simulink model "main_vehicle_v2"  (R2024b)
settings: Solver=FixedStepAuto  StartTime=0.0  StopTime=20  FixedStep=Ts  RelTol=1e-3
values from neighbouring files (symbols this model uses):
  Frr = Crr*m*g    (= 53.955)    [main_data_vehicle.m]
  v0 = 0.1    [main_data_vehicle.m]
undefined symbols (not defined in the file or in its folder): Sim3dSensor
libraries: sim3dlib x3, simulink x2, sim3dautolib x1, dspvision x1
settings Model: Creator=marti  LastModifiedBy=marti

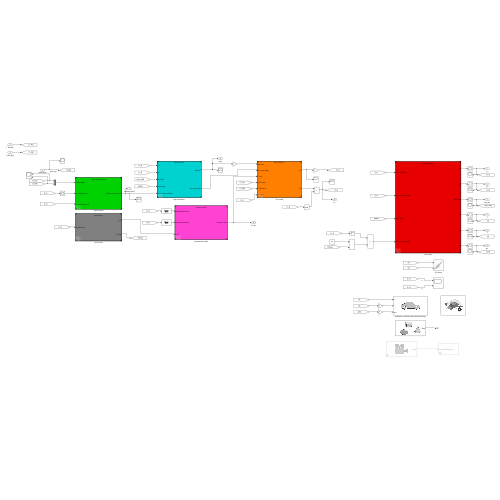
[thumbnail: Simulink's stored preview of the top-level diagram]
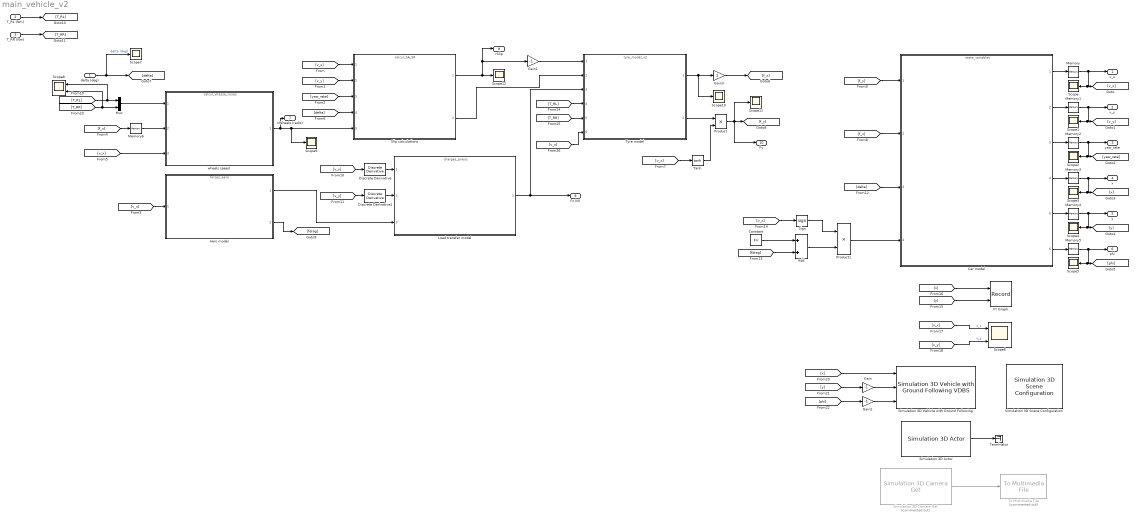
== system main_vehicle_v2 ==
  delta (deg) : Inport
  T_RL (Nm) : Inport  Port=2
  T_RR (Nm) : Inport  Port=3
  Add : Sum
  Aero model : ModelReference  ModelNameDialog=forces_aero.slx  SimulationMode=Normal  ModelReferenceVersion=1.5
  Car model : ModelReference  ModelNameDialog=state_variables.slx  SimulationMode=Normal  ModelReferenceVersion=1.11
  Constant : Constant  Value=Frr
  Discrete Derivative : simulink/Discrete/Discrete Derivative  gainval=1.0  ICPrevScaledInput=0.0  OutMin=[]  OutMax=[]  OutDataType=fixdt(1, 16)  OutScaling=2^-10  DoSatur=off
  Discrete Derivative1 : simulink/Discrete/Discrete Derivative  gainval=1.0  ICPrevScaledInput=0.0  OutMin=[]  OutMax=[]  OutDataType=fixdt(1, 16)  OutScaling=2^-10  DoSatur=off
  Gain : Gain  Gain=-1
  Gain1 : Gain  Gain=-1
  Gain2 : Gain  Gain=-1
  Gain3 : Gain
  Load transfer model : ModelReference  ModelNameDialog=charges_pneus.slx  SimulationMode=Normal  ModelReferenceVersion=1.22
  Memory : Memory  InitialCondition=v0
  Memory{1..5} (5 alike) : Memory
  Memory6 : Memory  InitialCondition=[0 0 0 0]
  Mux : Mux  Inputs=2
  Product : Product
  Product1 : Product
  Scope{,1..5,7,9..12} (11 alike) : Scope
  Scope6 : Scope  NumInputPorts=2
  Scope8 : Scope  NumInputPorts=2
  Sign : Signum
  Simulation 3D Actor : sim3dlib/Simulation 3D Actor  ActorName=Sim3dActor5  ParentName=Scene Origin  Operation=Create at setup  InitScriptText=skidpadConePlacement  SampleTime=.03  Translation=single([0 0 0])  Rotation=single([0 0 0])  Scale=single([1 1 1])  aMode=5  ActorTag=Sim3dActor5  ActorType=Sim3dActor  ID=5
      settings: LibrarySourceBlock=sl3dlib/Simulation 3D/Simulation 3D Actor
  Simulation 3D Camera Get : sim3dlib/Simulation 3D Camera Get  Priority=1  Commented=on  sensorTag=Sim3dSensor�  sensorId=2  sensorName=Sim3dSensor�  vehTagList={'Scene Origin';'Sim3dActor1';'Sim3dActor2';'Sim3dActor3';'Sim3dActor4';'Sim3dActor5';'SimulinkVehicle1'}  vehTag=SimulinkVehicle1  mountLoc=Origin  offsetFlag=on  tmountOffset=[-8, 0, 1]  rmountOffset=[0, 0, 0]  HorizontalResolution=1280  VerticalResolution=720  HorizontalFOV=60  SampleTime=0.03  mountPoint=[-8 0 1]  mountOrientation=[0 0 0]  aMode=5  ID=2
      settings: LibrarySourceBlock=sl3dlib/Simulation 3D/Utilities/Simulation 3D Camera Get
  Simulation 3D Scene Configuration : sim3dlib/Simulation 3D Scene Configuration  Priority=0  ProjectFormat=Default Scenes  SceneDesc=Straight road  ProjectName=C:\Program Files\MATLAB\R2024b\toolbox\shared\sim3d_projects\automotive_project_windows\UE\WindowsNoEditor\VehicleSimulation.exe  ScenePath=/Game/Maps/HwStrght  EnableOpenDRIVE=off  vehTagList={'Custom';'Scene Origin';'Sim3dActor1';'Sim3dActor2';'Sim3dActor3';'Sim3dActor4';'Sim3dActor5';'SimulinkVehicle1'}  vehTag=SimulinkVehicle1  FreeCameraInitialTranslation=[0, 0, 0]  FreeCameraDefaultInitialTranslation=[-6, 0, 2]  FreeCameraInitialRotation=[0, 0, 0]  FreeCameraDefaultInitialRotation=[0, -15, 0]  OpVisEn=off  Ts=.03  EnableWindow=on  EnableRemoteAccess=off  EnableWeather=off  SunAzimuth=90  SunAltitude=40.0  EnableGeospatialSun=off  Latitude=0  Longitude=0  Date=2023-01-01  Time=10:30:00  GeoTimeZone=-5.0  SunDaylightSaving=off  wind=1  clouds=10  EnableVolumetricClouds=off  CloudCoverage=0  CloudAltitude=6  fog=0  rain=0  RaindropsEffect=off  SnowDensity=0  EnableGeospatial=off  UseTrueOrigin=off  OriginHeight=200  OriginLatitude=40.744652  OriginLongitude=-73.988864  MapStyle=Aerial  AdditionalAssetIDs=[]  UseAdvancedSunSky=off  SolarTime=11  TimeZone=-5  Day=21  Month=9  Year=2022  UseDaylightSavingTime=on  DSTStartDay=10  DSTStartMonth=3  DSTEndDay=3  DSTEndMonth=11  DSTSwitchHour=2  sensorTag=MainCamera1  sensorId=1  sensorName=MainCamera1  mountLoc=Origin  offsetFlag=off  tmountOffset=[0, 0, 0]  rmountOffset=[0, 0, 0]  HorizontalResolution=1280  VerticalResolution=720  HorizontalFOV=60  mountPoint=[0 0 0]  mountOrientation=[0 0 0]  aMode=2  ID=1  GeoTrigger=Inactive
      settings: LibrarySourceBlock=vehdynlibsim3dcore/Simulation 3D Scene Configuration
  Simulation 3D Vehicle with Ground Following : sim3dautolib/Simulation 3D Vehicle with Ground Following VDBS  Priority=-1  PassVehMesh=Formula student vehicle  MeshPath=/MathWorksAutomotiveContent/Vehicles/Muscle/Meshes/SK_MuscleCar.SK_MuscleCar  TrackWidth=1.9  WheelBase=3  WheelRadius=0.35  VehColor=Silver  InitialPos=[0, 0, 0]  InitialRot=[0, 0, 0]  ActorName=SimulinkVehicle1  VehLightsControl=off  HeadlightColor=[ 1, 1, 1 ]  HighBeamIntensity=100000  LowBeamIntensity=60000  HighBeamConeAngle=1.22  LowBeamConeAngle=1.22  LeftHeadlightOrientation=[ 0, 0 ]  RightHeadlightOrientation=[ 0, 0 ]  BrakelightIntensity=200  ReverselightIntensity=500  SignallightIntensity=500  SignallightPeriod=1  SignalPulseWidth=50  SampleTime=-1  ActorType=SimulinkVehicle  ID=1  aMode=2  ActorTag=SimulinkVehicle1  CoordinateScheme=SAE
      settings: LibrarySourceBlock=vehdynlibsim3d/Simulation 3D Vehicle with Ground Following
  Slip calculations : ModelReference  ModelNameDialog=calcul_SA_SR.slx  SimulationMode=Normal  ModelReferenceVersion=1.30
  Tanh : Trigonometry  Operator=tanh
  Terminator : Terminator
  To Multimedia File : dspvision/To Multimedia File  Commented=on  outputFilename=C:\Users\marti\Documents\EPSA\Travaux torque structure\SKIDPAD.mp4  streamSelection=Video only  videoCompressor=None (uncompressed)  audioCompressor=None (uncompressed)  imagePorts=One multidimensional signal  fileType=MPEG4  audioDatatype=Determine from input data type  fourcc=RGB  audioBitRate=128  audioQuality=75  videoQuality=75  mj2000CompFactor=10
      settings: LibrarySourceBlock=visionsinks/To Multimedia File
  Tyre model : ModelReference  ModelNameDialog=tyre_model_v2.slx  SimulationMode=Normal  ModelReferenceVersion=1.15
  XY Graph : Record  FileSettingsInternal="{\"entries\":[{\"content\":{\"excelSettings\":{\"content\":{},\"type\":\"Streamout.ExcelSettings\"}},\"type\":\"Streamout.FileSettingStorage\",\"uuid\":\"\"}],\"packageUris\":[\"http:\\/\\/schema.mathworks.com\\/mf0\\/streamout_blocks\\/R2020a\"],\"version\":\"1.0\"}"  Layout=[1 1]  SignalsInternal="{\"entries\":[{\"content\":{\"signals\":[{\"content\":{\"blockPath\":[],\"dimensions\":[1],\"domain\":\"\",\"lineColor\":\"#edb120\",\"lineWidth\":2,\"port\":1,\"signalID\":1,\"signalName\":\"From16\"},\"type\":\"RecordBlkView.Signal\",\"uuid\":\"\"},{\"content\":{\"blockPath\":[],\"dimensions\":[1],\"domain\":\"\",\"lineColor\":\"#7e2f8e\",\"lineWidth\":2,\"port\":2,\"signalID\":2,\"signalName\":\"From15\"},\"type\":\"RecordBlkView.Signal\",\"uuid\":\"\"}]},\"type\":\"RecordBlkView.InputSignals\",\"uuid\":\"\"}],\"packageUris\":[\"http:\\/\\/schema.mathworks.com\\/mf0\\/streamout_blocks\\/R2020a\"],\"version\":\"1.0\"}"  VisualizationBindings="{\"xyplotplugin\":{\"info\":[{\"series\":[],\"subplotID\":1}]}}"  CompatibilityTag=XY
  wheels speed : ModelReference  ModelNameDialog=calcul_vitesse_roues.slx  SimulationMode=Normal  ModelReferenceVersion=1.37
  v_x : Outport
  v_y : Outport  Port=2
  yaw_rate : Outport  Port=3
  x : Outport  Port=4
  y : Outport  Port=5
  phi : Outport  Port=6
  nWheels (rad/s) : Outport  Port=7
  rSlip : Outport  Port=8
  Fz (N) : Outport  Port=9
  Fy : Outport  Port=10
  wires:
  Car model/1 -> Memory/1
  Car model/2 -> Memory1/1
  Car model/3 -> Memory2/1
  Car model/4 -> Memory3/1
  Car model/5 -> Memory4/1
  Car model/6 -> Memory5/1
  [v_x] -> Slip calculations/1
  [v_y] -> Slip calculations/2
  [yaw_rate] -> Slip calculations/3
  [v_x] -> Aero model/1
  [f_x] -> Memory6/1
  [delta] -> Slip calculations/4
  Memory/1 -> v_x/1, Scope/1, [v_x]
  Memory1/1 -> v_y/1, Scope1/1, [v_y]
  Memory2/1 -> yaw_rate/1, [yaw_rate], Scope2/1
  Memory3/1 -> x/1, Scope3/1, [x]
  Memory4/1 -> y/1, [y], Scope4/1
  Memory5/1 -> phi/1, Scope5/1, [phi]
  Mux/1 -> wheels speed/1
  [v_x] -> Discrete Derivative/1
  Discrete Derivative/1 -> Load transfer model/1
  [v_y] -> Discrete Derivative1/1
  Discrete Derivative1/1 -> Load transfer model/2
  wheels speed/1 -> nWheels (rad/s)/1, Scope9/1, Slip calculations/5
  [v_x] -> Tanh/1
  Tanh/1 -> Product/2
  [f_x] -> Car model/2
  [f_y] -> Car model/1
  [delta] -> Car model/3
  Aero model/1 -> Load transfer model/3
  Aero model/2 -> [fdrag]
  [fdrag] -> Add/2
  Constant/1 -> Add/1
  Product1/1 -> Car model/4
  Add/1 -> Product1/2
  Load transfer model/1 -> Fz (N)/1, Tyre model/3
  Tyre model/2 -> Product/1
  [v_x] -> Sign/1
  Sign/1 -> Product1/1
  delta (deg)/1 -> Scope7/1, [delta]  "delta (deg)"
  [y] -> XY Graph/2
  [x] -> XY Graph/1
  [v_x] -> Scope6/1  "v_x"
  [v_y] -> Scope6/2  "v_y"
  Product/1 -> Fy/1, Scope11/1, [f_y]
  Slip calculations/1 -> rSlip/1, Gain1/1, Scope12/1
  Slip calculations/2 -> Tyre model/2
  Gain1/1 -> Tyre model/1
  [v_x] -> wheels speed/3
  Memory6/1 -> wheels speed/2
  [x] -> Simulation 3D Vehicle with Ground Following/1
  [y] -> Gain/1
  [phi] -> Gain2/1
  Gain/1 -> Simulation 3D Vehicle with Ground Following/2
  Gain2/1 -> Simulation 3D Vehicle with Ground Following/3
  Simulation 3D Actor/1 -> Terminator/1
  Simulation 3D Camera Get/1 -> To Multimedia File/1
  T_RL (Nm)/1 -> [T_RL]
  T_RR (Nm)/1 -> [T_RR]
  [T_RR] -> Scope8/2, Mux/2
  [T_RL] -> Scope8/1, Mux/1
  [T_RL] -> Tyre model/4
  [T_RR] -> Tyre model/5
  Tyre model/1 -> Gain3/1, Scope10/1
  [v_x] -> Tyre model/6
  Gain3/1 -> [f_x]
